simulink model "no1_proportional_controller_22b"  (R2022b)
settings: Solver=VariableStepAuto  StartTime=0.0  StopTime=50  RelTol=1e-3
settings Model: Creator=ayeo  LastModifiedBy=ayeo
settings OptimizationCC: ReuseModelBlockBuffer=on
settings RTWCC: GPUComputeCapability=5.0
settings ConfigComp: CovBoundaryAbsTol=1.0e-5

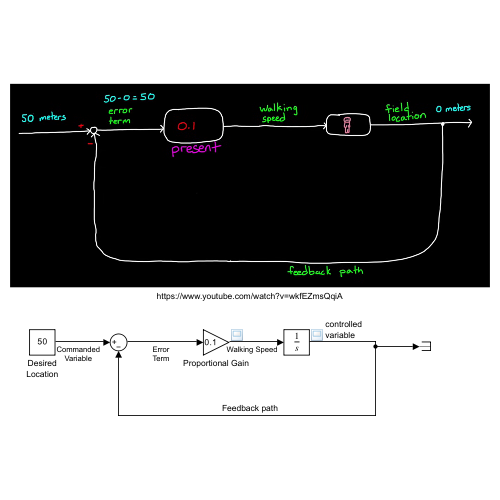
[thumbnail: Simulink's stored preview of the top-level diagram]
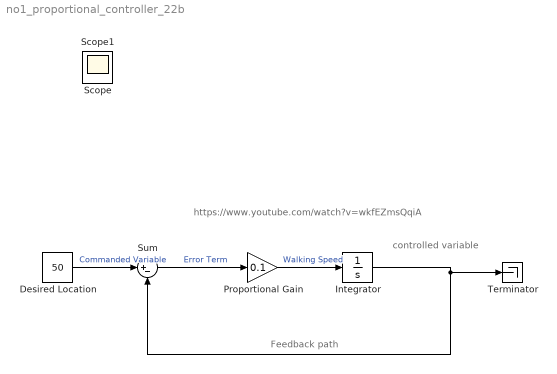
== system no1_proportional_controller_22b ==
  note: https://www.youtube.com/watch?v=wkfEZmsQqiA
  note: controlled
      | variable
  note: Feedback path
  Desired Location : Constant  Value=50
  Integrator : Integrator
  Proportional Gain : Gain  Gain=0.1
  Sum : Sum  Inputs=|+-
  Terminator : Terminator
  Scope : Scope
  Scope1 : Scope
  wires:
  Desired Location/1 -> Sum/1  "Commanded Variable"
  Sum/1 -> Proportional Gain/1  "Error Term"
  Proportional Gain/1 -> Integrator/1  "Walking Speed"
  Integrator/1 -> Sum/2, Terminator/1
